simulink model "BASIC_PRACTICES"  (R2025a)
settings: Solver=FixedStepDiscrete  StartTime=0.0  StopTime=10.0  FixedStep=.5  RelTol=1e-3
libraries: simulink x15, simulink_extras x1, SignalEditorBlockLib x1
settings Model: Creator=shubh  LastModifiedBy=shubh

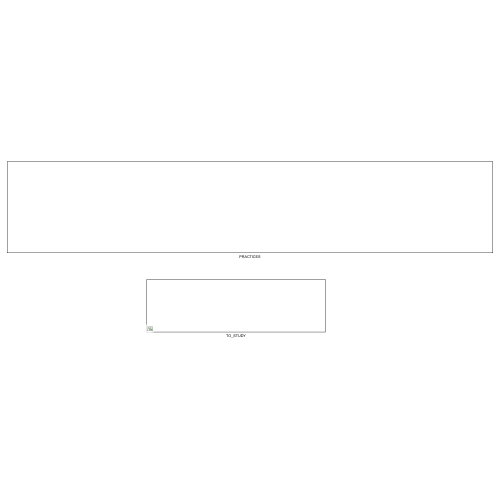
[thumbnail: Simulink's stored preview of the top-level diagram]
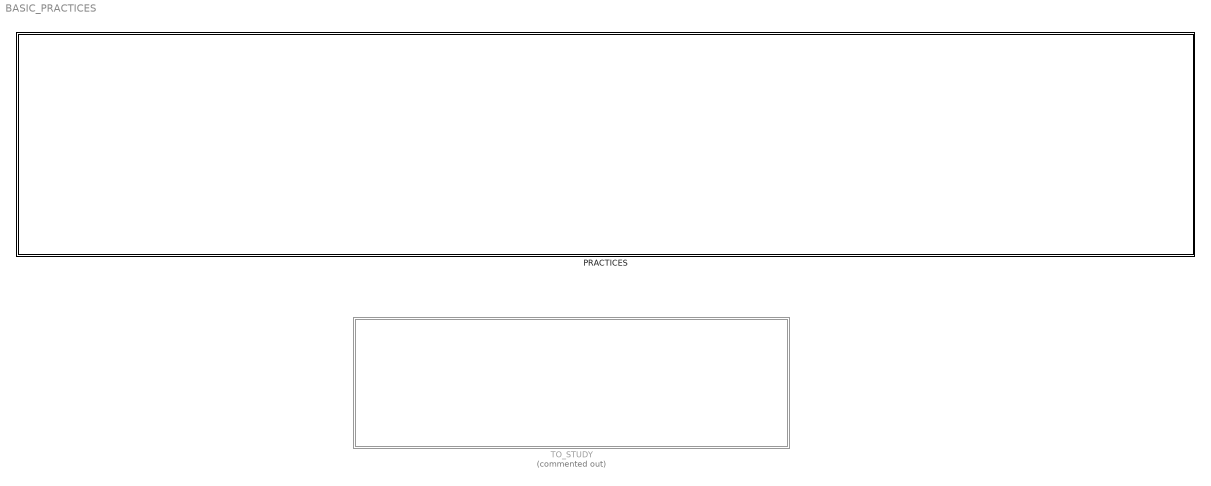
== system BASIC_PRACTICES ==
  PRACTICES : Subsystem
  TO_STUDY : Subsystem  Commented=on

== system BASIC_PRACTICES/PRACTICES ==
  Simulink : Subsystem  Commented=on
  Stateflow : Subsystem  Commented=on
  Subsystem : Subsystem  Commented=on

== system BASIC_PRACTICES/TO_STUDY ==
  Chart : Stateflow chart  TreatAsAtomicUnit=on
  Signal Editor : SignalEditorBlockLib/Signal Editor  FileName=untitled.mat  ActiveScenario=Scenario  ActiveSignal=Signal 1  IsBus=off  OutputBusObjectStr=Bus: BusObject  SampleTime=0  Interpolate=off  ZeroCross=off  OutputAfterFinalValue=Setting to zero  Unit=inherit  PreserveSignalName=on  ApplySigPropsToAllScenarios=on  ApplySigPropsToAllSignals=off  SignalPropertySource=Dialog parameters

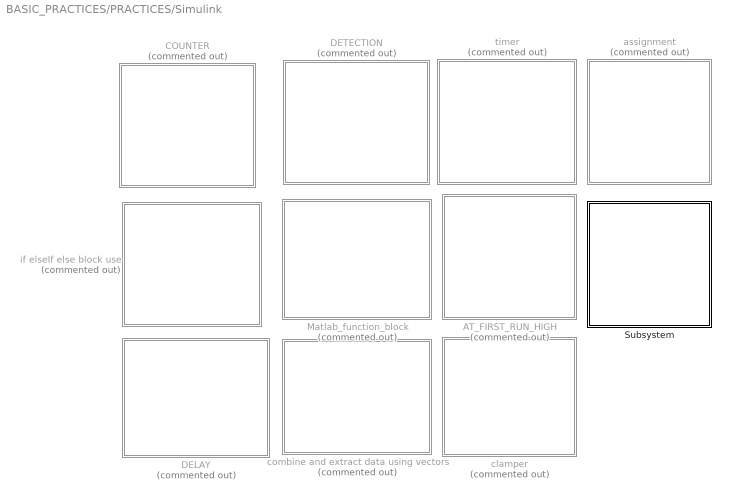
== system BASIC_PRACTICES/PRACTICES/Simulink ==
  AT_FIRST_RUN_HIGH : Subsystem  Commented=on
  COUNTER : Subsystem  Commented=on
  DELAY : Subsystem  Commented=on
  DETECTION : Subsystem  Commented=on
  Matlab_function_block : Subsystem  Commented=on
  Subsystem : Subsystem
  assignment : Subsystem  Commented=on
  clamper : Subsystem  Commented=on
  combine and extract data using vectors : Subsystem  Commented=on
  if elseIf else block use : Subsystem  Commented=on
  timer : Subsystem  Commented=on

== system BASIC_PRACTICES/PRACTICES/Stateflow ==
  For_loop : Subsystem  Commented=on
  counter : Subsystem  Commented=on
  delay_wo_delay_block : Subsystem  Commented=on
  if_else : Subsystem  Commented=on

== system BASIC_PRACTICES/PRACTICES/Subsystem ==
  BY_MATLAB_function : Subsystem  Commented=on
  Subsystem : Subsystem

== system BASIC_PRACTICES/TO_STUDY/Chart/? ==
  Action Port : ActionPort
      settings: CopyFcn=Stateflow.SLINSF.SimulinkMan.removeBlockPreDeleteFcn  PreDeleteFcn=Stateflow.SLINSF.SimulinkMan.unsafePredeleteFcn

== system BASIC_PRACTICES/TO_STUDY/Chart/?1 ==
  Action Port : ActionPort
      settings: CopyFcn=Stateflow.SLINSF.SimulinkMan.removeBlockPreDeleteFcn  PreDeleteFcn=Stateflow.SLINSF.SimulinkMan.unsafePredeleteFcn

== system BASIC_PRACTICES/TO_STUDY/Chart/?2 ==
  f : TriggerPort  TriggerType=function-call  VariantControl=(inherit)
      settings: CopyFcn=Stateflow.SLINSF.SimulinkMan.removeBlockPreDeleteFcn  PreDeleteFcn=Stateflow.SLINSF.SimulinkMan.unsafePredeleteFcn

== system BASIC_PRACTICES/PRACTICES/Simulink/AT_FIRST_RUN_HIGH ==
  AND : Logic  IconShape=distinctive  AllPortsSameDT=off  OutDataTypeStr=boolean
  Constant : Constant  OutDataTypeStr=boolean
  Pulse Generator : DiscretePulseGenerator  PulseType=Time based  Amplitude=2  PulseWidth=50  PhaseDelay=1
  Scope : Scope  NumInputPorts=2
      settings: ActiveDisplayYMinimum=-1  ActiveDisplayYMaximum=1
  Switch : Switch  Criteria=u2 > Threshold  SaturateOnIntegerOverflow=off  InputSameDT=off
  Unit Delay : UnitDelay  SampleTime=-1  HasFrameUpgradeWarning=on
  wires:
  Constant/1 -> AND/1
  Switch/1 -> Unit Delay/1, Scope/1
  Pulse Generator/1 -> Scope/2, AND/2
  AND/1 -> Switch/1, Switch/2
  Unit Delay/1 -> Switch/3

== system BASIC_PRACTICES/PRACTICES/Simulink/COUNTER ==
  DOWN : Subsystem
  UP_DOWN : Subsystem
  enabled_and_reset : Subsystem
  up : Subsystem

== system BASIC_PRACTICES/PRACTICES/Simulink/DELAY ==
  OFF_DELAY_WITH_BASIC_BLOCKS : Subsystem
  ON_DELAY_WITH_BASIC_BLOCKS : Subsystem
  ON_OFF_DELAY_ONE_STEP : Subsystem

== system BASIC_PRACTICES/PRACTICES/Simulink/DETECTION ==
  EDGE_DETECTION : Subsystem
  HYSTERESIS : Subsystem
  OUT_OF_RANGE_DETECTION : Subsystem
  max-of-three-input : Subsystem

== system BASIC_PRACTICES/PRACTICES/Simulink/Matlab_function_block ==
  MATLAB Function : MATLAB Function  TreatAsAtomicUnit=on
  Repeating Sequence Stair : simulink/Sources/Repeating Sequence Stair  OutValues=[1 -2 2 3].'  tsamp=-1  OutMin=[]  OutMax=[]  OutDataTypeStr=double  OutputDataTypeScalingMode=double  OutDataType=fixdt(0,8)  ConRadixGroup=Best Precision: Vector-wise  OutScaling=2^-12
  Scope : Scope  NumInputPorts=2
      settings: ActiveDisplayYMinimum=-2.625  ActiveDisplayYMaximum=3.625  DataLoggingVariableName=ScopeData2
  wires:
  MATLAB Function/1(y) -> Scope/2
  Repeating Sequence Stair/1 -> Scope/1, MATLAB Function/1(u)

== system BASIC_PRACTICES/PRACTICES/Simulink/Subsystem ==

== system BASIC_PRACTICES/PRACTICES/Simulink/assignment ==
  Assignment : Assignment  DiagnosticForDimensions=Warning  IndexOptions=Starting index (port)  Indices=[2 ]  OutputSizes=5
  Constant : Constant  Value=[0 0 0 0 0]
  Display : Display
  Repeating Sequence Stair : simulink/Sources/Repeating Sequence Stair  OutValues=[5 4 3 2 1].'  tsamp=-1  OutMin=[]  OutMax=[]  OutDataTypeStr=double  OutputDataTypeScalingMode=double  OutDataType=fixdt(0,8)  ConRadixGroup=Best Precision: Vector-wise  OutScaling=2^-12
  Repeating Sequence Stair1 : simulink/Sources/Repeating Sequence Stair  OutValues=[1 2 3 4 5].'  tsamp=-1  OutMin=[]  OutMax=[]  OutDataTypeStr=double  OutputDataTypeScalingMode=double  OutDataType=fixdt(0,8)  ConRadixGroup=Best Precision: Vector-wise  OutScaling=2^-12
  wires:
  Constant/1 -> Assignment/1
  Repeating Sequence Stair/1 -> Assignment/2
  Assignment/1 -> Display/1
  Repeating Sequence Stair1/1 -> Assignment/3

== system BASIC_PRACTICES/PRACTICES/Simulink/clamper ==
  Add : Sum
  Constant : Constant
  Repeating Sequence Stair : simulink/Sources/Repeating Sequence Stair  OutValues=[-5 5].'  tsamp=-1  OutMin=[]  OutMax=[]  OutDataTypeStr=double  OutputDataTypeScalingMode=double  OutDataType=fixdt(0,8)  ConRadixGroup=Best Precision: Vector-wise  OutScaling=2^-12
  Scope : Scope  NumInputPorts=2
      settings: ActiveDisplayYMinimum=-6.25  ActiveDisplayYMaximum=6.25  DataLoggingVariableName=ScopeData2
  wires:
  Add/1 -> Scope/2
  Repeating Sequence Stair/1 -> Scope/1, Add/1
  Constant/1 -> Add/2

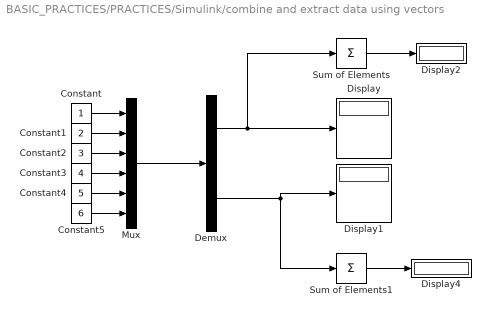
== system BASIC_PRACTICES/PRACTICES/Simulink/combine and extract data using vectors ==
  Constant : Constant
  Constant1 : Constant  Value=2
  Constant2 : Constant  Value=3
  Constant3 : Constant  Value=4
  Constant4 : Constant  Value=5
  Constant5 : Constant  Value=6
  Demux : Demux  Outputs=2
  Display{,1..2,4} (4 alike) : Display
  Mux : Mux  Inputs=6
  Sum of Elements : Sum  Inputs=+
  Sum of Elements1 : Sum  Inputs=+
  wires:
  Mux/1 -> Demux/1
  Constant5/1 -> Mux/6
  Constant4/1 -> Mux/5
  Constant3/1 -> Mux/4
  Constant2/1 -> Mux/3
  Constant1/1 -> Mux/2
  Constant/1 -> Mux/1
  Demux/1 -> Sum of Elements/1, Display/1
  Demux/2 -> Display1/1, Sum of Elements1/1
  Sum of Elements/1 -> Display2/1
  Sum of Elements1/1 -> Display4/1

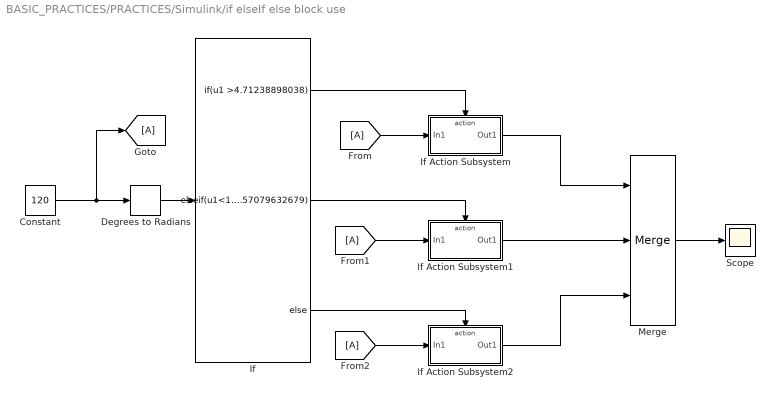
== system BASIC_PRACTICES/PRACTICES/Simulink/if elseIf else block use ==
  Constant : Constant  Value=120  OutDataTypeStr=Inherit: Inherit via back propagation
  Degrees to Radians : simulink_extras/Transformations/Degrees to Radians
  From : From
  From1 : From
  From2 : From
  Goto : Goto
  If : If  IfExpression=u1 >4.71238898038  ElseIfExpressions=u1<1.57079632679
  If Action Subsystem : Subsystem  TreatAsAtomicUnit=on
  If Action Subsystem1 : Subsystem  TreatAsAtomicUnit=on
  If Action Subsystem2 : Subsystem  TreatAsAtomicUnit=on
  Merge : Merge  Inputs=3
  Scope : Scope
      settings: ActiveDisplayYMinimum=0.48061  ActiveDisplayYMaximum=0.68061
  wires:
  Constant/1 -> Degrees to Radians/1, Goto/1
  Merge/1 -> Scope/1
  From/1 -> If Action Subsystem/1(In1)
  From1/1 -> If Action Subsystem1/1(In1)
  From2/1 -> If Action Subsystem2/1(In1)
  If/3 -> If Action Subsystem2/Action
  If/2 -> If Action Subsystem1/Action
  If/1 -> If Action Subsystem/Action
  If Action Subsystem/1(Out1) -> Merge/1
  If Action Subsystem1/1(Out1) -> Merge/2
  If Action Subsystem2/1(Out1) -> Merge/3
  Degrees to Radians/1 -> If/1

== system BASIC_PRACTICES/PRACTICES/Simulink/timer ==
  Counting_1_MINUTE : Subsystem  Commented=on
  OFF_DELAY_WITH_BASIC_BLOCKS : Subsystem  Commented=on
  ON_DELAY_WITH_BASIC_BLOCKS : Subsystem  Commented=on
  ON_OFF_DELAY_ONE_STEP : Subsystem  Commented=on

== system BASIC_PRACTICES/PRACTICES/Stateflow/For_loop ==
  Chart : Stateflow chart  TreatAsAtomicUnit=on
  Chart1 : Stateflow chart  TreatAsAtomicUnit=on
  Repeating Sequence Stair : simulink/Sources/Repeating Sequence Stair  OutValues=[0 1].'  tsamp=-1  OutMin=[]  OutMax=[]  OutDataTypeStr=double  OutputDataTypeScalingMode=double  OutDataType=fixdt(0,8)  ConRadixGroup=Best Precision: Vector-wise  OutScaling=2^-12
  Scope : Scope  NumInputPorts=2
      settings: ActiveDisplayYMinimum=45  ActiveDisplayYMaximum=65  DataLoggingVariableName=ScopeData2
  wires:
  Chart1/1(out) -> Scope/1
  Chart/1(out) -> Scope/2
  Repeating Sequence Stair/1 -> Chart/1(en)

== system BASIC_PRACTICES/PRACTICES/Stateflow/counter ==
  Chart : Stateflow chart  TreatAsAtomicUnit=on
  Scope : Scope
      settings: ActiveDisplayYMinimum=-0.625  ActiveDisplayYMaximum=5.625  DataLoggingVariableName=ScopeData4
  wires:
  Chart/1(z) -> Scope/1

== system BASIC_PRACTICES/PRACTICES/Stateflow/delay_wo_delay_block ==
  Chart : Stateflow chart  TreatAsAtomicUnit=on
      settings: PortSchema="{\"entries\":[{\"content\":{\"sides\":[{\"content\":{\"connectorIds\":[\"In4\",\"In1\",\"In2\",\"In3\"]},\"type\":\"ConnectorPlacement.EquallySpacedRectSide\",\"uuid\":\"e0e5e045-d7b2-46b3-b410-3be38740735a\"},{\"content\":{\"connectorIds\":[\"Out1\",\"Out2\"],\"side\":\"RIGHT\"},\"type\":\"ConnectorPlacement.EquallySpacedRectSide\",\"uuid\":\"4f12564d-9a97-4df6-80a9-b07c0bfc5d80\"},{\"content\":{\"side\":\"TOP\"},\"type\":\"ConnectorPlacement.EquallySpacedRectSide\",\"uuid\":\"29280d5c-fd79-4991-91bd-bd3cbc2b5a83\"}]},\"type\":\"ConnectorPlacement.EquallySpacedConnector\",\"uuid\":\"51515ad8-eb0a-4d19-8f24-8c6bcb3a19d7\"}],\"packageUris\":[\"http://schema.mathworks.com/mf0/Connector/R2020b\"],\"version\":\"1.0\"}"
  Constant : Constant  OutDataTypeStr=uint16
  Counter Free-Running : simulink/Sources/Counter Free-Running  NumBits=16  tsamp=-1
  Data Store Memory : DataStoreMemory  WriteAfterWriteMsg=warning  ShowAdditionalParam=off
  Data Store Read : DataStoreRead  IndexOptions=Index vector (dialog)  Indices=1  OutputSizes=1
  Data Store Write1 : DataStoreWrite  IndexOptions=Index vector (dialog)  Indices=1  OutputSizes=1
  Repeating Sequence Stair : simulink/Sources/Repeating Sequence Stair  OutValues=[3 1 2].'  tsamp=-1  OutMin=[]  OutMax=[]  OutDataTypeStr=uint16  OutputDataTypeScalingMode=uint16  OutDataType=fixdt(0,8)  ConRadixGroup=Best Precision: Vector-wise  OutScaling=2^-12
  Scope : Scope  NumInputPorts=3
      settings: ActiveDisplayYMinimum=0.75  ActiveDisplayYMaximum=3.25
  wires:
  Counter Free-Running/1 -> Chart/3(t)
  Repeating Sequence Stair/1 -> Chart/4(in), Scope/1
  Constant/1 -> Chart/1(inVal)
  Data Store Read/1 -> Chart/2(oldIn)
  Chart/2(oldValue) -> Scope/3, Data Store Write1/1
  Chart/1(out) -> Scope/2

== system BASIC_PRACTICES/PRACTICES/Stateflow/if_else ==
  Chart : Stateflow chart  TreatAsAtomicUnit=on
  Constant : Constant
  Scope : Scope
      settings: DataLoggingVariableName=ScopeData3
  wires:
  Chart/1(y) -> Scope/1
  Constant/1 -> Chart/1(h)

== system BASIC_PRACTICES/PRACTICES/Subsystem/BY_MATLAB_function ==
  Constant : Constant  Value=5
  Display : Display
  MATLAB Function : MATLAB Function  TreatAsAtomicUnit=on
  wires:
  Constant/1 -> MATLAB Function/1(n)
  MATLAB Function/1(y) -> Display/1

== system BASIC_PRACTICES/PRACTICES/Subsystem/Subsystem ==
  note: run 1 step for correct
      | output
  Constant : Constant  Value=5
  Display : Display
  For Iterator Subsystem : Subsystem  TreatAsAtomicUnit=on
  wires:
  Constant/1 -> For Iterator Subsystem/1(In2)
  For Iterator Subsystem/1(Out1) -> Display/1

== system BASIC_PRACTICES/PRACTICES/Simulink/COUNTER/DOWN ==
  Add : Sum  Inputs=-+
  Compare To Constant : simulink/Logic and Bit Operations/Compare To Constant  relop=<=  const=0  OutDataTypeStr=boolean
  Constant : Constant
  Constant2 : Constant  Value=5
  Scope : Scope
      settings: ActiveDisplayYMinimum=-24.56203  ActiveDisplayYMaximum=9.14991
  Switch : Switch  Criteria=u2 > Threshold  SaturateOnIntegerOverflow=off  InputSameDT=off
  Unit Delay : UnitDelay  InitialCondition=6  SampleTime=-1  HasFrameUpgradeWarning=on
  wires:
  Constant/1 -> Add/1
  Add/1 -> Switch/3, Compare To Constant/1
  Unit Delay/1 -> Add/2
  Switch/1 -> Unit Delay/1, Scope/1
  Compare To Constant/1 -> Switch/2
  Constant2/1 -> Switch/1

== system BASIC_PRACTICES/PRACTICES/Simulink/COUNTER/UP_DOWN ==

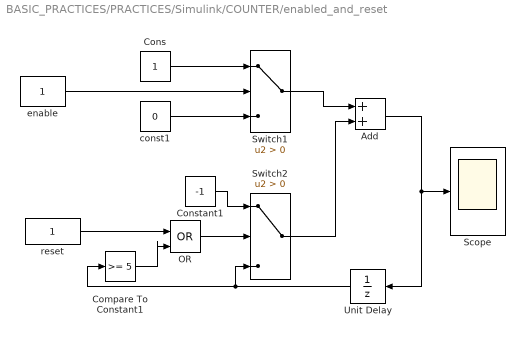
== system BASIC_PRACTICES/PRACTICES/Simulink/COUNTER/enabled_and_reset ==
  Add : Sum
  Compare To Constant1 : simulink/Logic and Bit Operations/Compare To Constant  relop=>=  const=5  OutDataTypeStr=boolean
  Cons : Constant
  Constant1 : Constant  Value=-1
  OR : Logic  Operator=OR  IconShape=distinctive  AllPortsSameDT=off  OutDataTypeStr=boolean
  Scope : Scope
      settings: ActiveDisplayYMinimum=-0.625  ActiveDisplayYMaximum=5.625
  Switch1 : Switch  Criteria=u2 > Threshold  SaturateOnIntegerOverflow=off  InputSameDT=off
  Switch2 : Switch  Criteria=u2 > Threshold  SaturateOnIntegerOverflow=off  InputSameDT=off
  Unit Delay : UnitDelay  InitialCondition=-1  SampleTime=-1  HasFrameUpgradeWarning=on
  const1 : Constant  Value=0
  enable : Constant
  reset : Constant
  wires:
  Add/1 -> Unit Delay/1, Scope/1
  Unit Delay/1 -> Compare To Constant1/1, Switch2/3
  Switch1/1 -> Add/1
  const1/1 -> Switch1/3
  Cons/1 -> Switch1/1
  enable/1 -> Switch1/2
  Switch2/1 -> Add/2
  reset/1 -> OR/1
  Constant1/1 -> Switch2/1
  Compare To Constant1/1 -> OR/2
  OR/1 -> Switch2/2

== system BASIC_PRACTICES/PRACTICES/Simulink/COUNTER/up ==
  Add : Sum
  Compare To Constant : simulink/Logic and Bit Operations/Compare To Constant  relop=<=  const=5  OutDataTypeStr=boolean
  Constant : Constant
  Constant1 : Constant  Value=0
  Scope1 : Scope
      settings: ActiveDisplayYMinimum=-0.625  ActiveDisplayYMaximum=5.625  DataLoggingVariableName=ScopeData2
  Switch : Switch  Criteria=u2 > Threshold  SaturateOnIntegerOverflow=off  InputSameDT=off
  Unit Delay : UnitDelay  InitialCondition=-1  SampleTime=-1  HasFrameUpgradeWarning=on
  wires:
  Switch/1 -> Scope1/1, Unit Delay/1
  Add/1 -> Switch/1, Compare To Constant/1
  Compare To Constant/1 -> Switch/2
  Constant/1 -> Add/1
  Constant1/1 -> Switch/3
  Unit Delay/1 -> Add/2

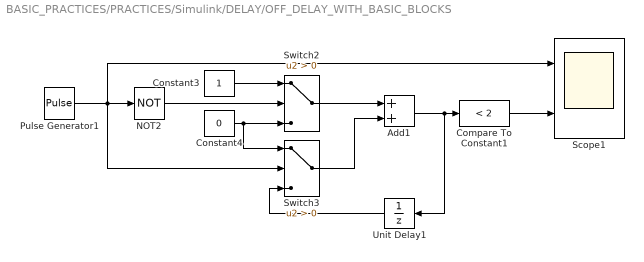
== system BASIC_PRACTICES/PRACTICES/Simulink/DELAY/OFF_DELAY_WITH_BASIC_BLOCKS ==
  Add1 : Sum
  Compare To Constant1 : simulink/Logic and Bit Operations/Compare To Constant  relop=<  const=2  OutDataTypeStr=boolean
  Constant3 : Constant
  Constant4 : Constant  Value=0
  NOT2 : Logic  Operator=NOT  IconShape=distinctive  AllPortsSameDT=off  OutDataTypeStr=boolean
  Pulse Generator1 : DiscretePulseGenerator  PulseType=Time based  PulseWidth=50  PhaseDelay=.5
  Scope1 : Scope  NumInputPorts=2
      settings: ActiveDisplayYMinimum=-0.125  ActiveDisplayYMaximum=1.125  DataLoggingVariableName=ScopeData3
  Switch2 : Switch  Criteria=u2 > Threshold  SaturateOnIntegerOverflow=off  InputSameDT=off
  Switch3 : Switch  Criteria=u2 > Threshold  SaturateOnIntegerOverflow=off  InputSameDT=off
  Unit Delay1 : UnitDelay  SampleTime=-1  HasFrameUpgradeWarning=on
  wires:
  Switch3/1 -> Add1/2
  NOT2/1 -> Switch2/2
  Unit Delay1/1 -> Switch3/3
  Add1/1 -> Unit Delay1/1, Compare To Constant1/1
  Compare To Constant1/1 -> Scope1/2
  Constant4/1 -> Switch3/1, Switch2/3
  Pulse Generator1/1 -> Switch3/2, NOT2/1, Scope1/1
  Constant3/1 -> Switch2/1
  Switch2/1 -> Add1/1

== system BASIC_PRACTICES/PRACTICES/Simulink/DELAY/ON_DELAY_WITH_BASIC_BLOCKS ==
  note: RISING_DELAY_0.5sec_SOLVER=.25
  Add1 : Sum
  Compare To Constant1 : simulink/Logic and Bit Operations/Compare To Constant  relop=>=  const=.75  OutDataTypeStr=boolean
  Constant3 : Constant  Value=.25
  Constant4 : Constant  Value=0
  NOT1 : Logic  Operator=NOT  IconShape=distinctive  AllPortsSameDT=off  OutDataTypeStr=boolean
  Pulse Generator1 : DiscretePulseGenerator  PulseType=Time based  PulseWidth=50  PhaseDelay=.5
  Scope1 : Scope  NumInputPorts=2
      settings: ActiveDisplayYMinimum=-0.125  ActiveDisplayYMaximum=1.125  DataLoggingVariableName=ScopeData6
  Switch2 : Switch  Criteria=u2 > Threshold  SaturateOnIntegerOverflow=off  InputSameDT=off
  Switch3 : Switch  Criteria=u2 > Threshold  SaturateOnIntegerOverflow=off  InputSameDT=off
  Unit Delay1 : UnitDelay  SampleTime=-1  HasFrameUpgradeWarning=on
  wires:
  NOT1/1 -> Switch3/2
  Switch3/1 -> Add1/2
  Constant3/1 -> Switch2/1
  Switch2/1 -> Add1/1
  Add1/1 -> Unit Delay1/1, Compare To Constant1/1
  Compare To Constant1/1 -> Scope1/2
  Unit Delay1/1 -> Switch3/3
  Pulse Generator1/1 -> NOT1/1, Switch2/2, Scope1/1
  Constant4/1 -> Switch3/1, Switch2/3

== system BASIC_PRACTICES/PRACTICES/Simulink/DELAY/ON_OFF_DELAY_ONE_STEP ==
  OFF_DELAY : Subsystem  Commented=on
  ON_DELAY : Subsystem  Commented=on

== system BASIC_PRACTICES/PRACTICES/Simulink/DETECTION/EDGE_DETECTION ==
  FALLING : Subsystem  Commented=on
  FALLING_EDGE_COUNT : Subsystem  Commented=on
  Rising : Subsystem  Commented=on
  Rising_EDGE_COUNT : Subsystem  Commented=on
  rising_falling_edge_detection_and_counting : Subsystem  Commented=on

== system BASIC_PRACTICES/PRACTICES/Simulink/DETECTION/HYSTERESIS ==
  BLOCK : Subsystem  Commented=on
  HYSTERESIS : Subsystem  Commented=on
  REVERSE_HYSTERESIS : Subsystem  Commented=on

== system BASIC_PRACTICES/PRACTICES/Simulink/DETECTION/OUT_OF_RANGE_DETECTION ==
  AND1 : Logic  Operator=OR  IconShape=distinctive  AllPortsSameDT=off  OutDataTypeStr=boolean
  Constant : Constant  Value=2
  Constant1 : Constant  Value=-2
  Constant2 : Constant  OutDataTypeStr=boolean
  Constant3 : Constant  Value=0  OutDataTypeStr=boolean
  GreaterThan : RelationalOperator  Operator=>  OutDataTypeStr=boolean  RndMeth=Simplest  InputSameDT=off
  GreaterThan1 : RelationalOperator  Operator=<  OutDataTypeStr=boolean  RndMeth=Simplest  InputSameDT=off
  Scope1 : Scope  NumInputPorts=2
      settings: ActiveDisplayYMinimum=-3.73705  ActiveDisplayYMaximum=3.74854
  Sine Wave1 : Sin  Amplitude=3  Frequency=3  SampleTime=0
  Switch : Switch  Criteria=u2 > Threshold  SaturateOnIntegerOverflow=off  InputSameDT=off
  wires:
  GreaterThan1/1 -> AND1/2
  Sine Wave1/1 -> GreaterThan1/1, GreaterThan/1, Scope1/1
  Constant/1 -> GreaterThan/2
  Constant3/1 -> Switch/3
  Constant1/1 -> GreaterThan1/2
  GreaterThan/1 -> AND1/1
  AND1/1 -> Switch/2
  Constant2/1 -> Switch/1
  Switch/1 -> Scope1/2

== system BASIC_PRACTICES/PRACTICES/Simulink/DETECTION/max-of-three-input ==
  A : Constant  Value=56
  B : Constant  Value=45
  C : Constant  Value=46
  Display1 : Display
  GreaterThan : RelationalOperator  Operator=>  OutDataTypeStr=boolean  RndMeth=Simplest  InputSameDT=off
  GreaterThanC : RelationalOperator  Operator=>  OutDataTypeStr=boolean  RndMeth=Simplest  InputSameDT=off
  Switch : Switch  Criteria=u2 > Threshold  SaturateOnIntegerOverflow=off  InputSameDT=off
  Switch1 : Switch  Criteria=u2 > Threshold  SaturateOnIntegerOverflow=off  InputSameDT=off
  wires:
  B/1 -> GreaterThan/2, Switch/3
  A/1 -> GreaterThan/1, Switch/1
  GreaterThan/1 -> Switch/2
  Switch/1 -> GreaterThanC/1, Switch1/1
  C/1 -> GreaterThanC/2, Switch1/3
  GreaterThanC/1 -> Switch1/2
  Switch1/1 -> Display1/1

== system BASIC_PRACTICES/PRACTICES/Simulink/if elseIf else block use/If Action Subsystem ==
  In1 : Inport
  Action Port : ActionPort  ActionPortLabel=if(u1 >4.71238898038)
  Multiply : Gain  Gain=0
  Out1 : Outport
  wires:
  In1/1 -> Multiply/1
  Multiply/1 -> Out1/1

== system BASIC_PRACTICES/PRACTICES/Simulink/if elseIf else block use/If Action Subsystem1 ==
  In1 : Inport
  Action Port : ActionPort  ActionPortLabel=elseif(u1<1.57079632679)
  Multiply : Gain  Gain=0
  Out1 : Outport
  wires:
  In1/1 -> Multiply/1
  Multiply/1 -> Out1/1

== system BASIC_PRACTICES/PRACTICES/Simulink/if elseIf else block use/If Action Subsystem2 ==
  In1 : Inport
  Action Port : ActionPort  ActionPortLabel=else
  Sinh1 : Trigonometry
  Out1 : Outport
  wires:
  Sinh1/1 -> Out1/1
  In1/1 -> Sinh1/1

== system BASIC_PRACTICES/PRACTICES/Simulink/timer/Counting_1_MINUTE ==
  Add1 : Sum
  Constant2 : Constant
  Constant3 : Constant  Value=61
  GreaterThan1 : RelationalOperator  Operator===  OutDataTypeStr=boolean  RndMeth=Simplest  InputSameDT=off
  Scope1 : Scope
      settings: ActiveDisplayYMinimum=-0.125  ActiveDisplayYMaximum=1.125  DataLoggingVariableName=ScopeData6
  Unit Delay1 : UnitDelay  SampleTime=-1  HasFrameUpgradeWarning=on
  wires:
  Add1/1 -> Unit Delay1/1, GreaterThan1/1
  GreaterThan1/1 -> Scope1/1
  Constant2/1 -> Add1/1
  Unit Delay1/1 -> Add1/2
  Constant3/1 -> GreaterThan1/2

== system BASIC_PRACTICES/PRACTICES/Simulink/timer/OFF_DELAY_WITH_BASIC_BLOCKS ==
  Add1 : Sum
  Compare To Constant1 : simulink/Logic and Bit Operations/Compare To Constant  relop=<  const=2  OutDataTypeStr=boolean
  Constant3 : Constant
  Constant4 : Constant  Value=0
  NOT2 : Logic  Operator=NOT  IconShape=distinctive  AllPortsSameDT=off  OutDataTypeStr=boolean
  Pulse Generator1 : DiscretePulseGenerator  PulseType=Time based  PulseWidth=50  PhaseDelay=.5
  Scope1 : Scope  NumInputPorts=2
      settings: ActiveDisplayYMinimum=-0.125  ActiveDisplayYMaximum=1.125  DataLoggingVariableName=ScopeData3
  Switch2 : Switch  Criteria=u2 > Threshold  SaturateOnIntegerOverflow=off  InputSameDT=off
  Switch3 : Switch  Criteria=u2 > Threshold  SaturateOnIntegerOverflow=off  InputSameDT=off
  Unit Delay1 : UnitDelay  SampleTime=-1  HasFrameUpgradeWarning=on
  wires:
  Switch3/1 -> Add1/2
  NOT2/1 -> Switch2/2
  Unit Delay1/1 -> Switch3/3
  Add1/1 -> Unit Delay1/1, Compare To Constant1/1
  Compare To Constant1/1 -> Scope1/2
  Constant4/1 -> Switch3/1, Switch2/3
  Pulse Generator1/1 -> Switch3/2, NOT2/1, Scope1/1
  Constant3/1 -> Switch2/1
  Switch2/1 -> Add1/1

== system BASIC_PRACTICES/PRACTICES/Simulink/timer/ON_DELAY_WITH_BASIC_BLOCKS ==
  note: RISING_DELAY_0.5sec_SOLVER=.25
  Add1 : Sum
  Compare To Constant1 : simulink/Logic and Bit Operations/Compare To Constant  relop=>=  const=.75  OutDataTypeStr=boolean
  Constant3 : Constant  Value=.25
  Constant4 : Constant  Value=0
  NOT1 : Logic  Operator=NOT  IconShape=distinctive  AllPortsSameDT=off  OutDataTypeStr=boolean
  Pulse Generator1 : DiscretePulseGenerator  PulseType=Time based  PulseWidth=50  PhaseDelay=.5
  Scope1 : Scope  NumInputPorts=2
      settings: ActiveDisplayYMinimum=-0.125  ActiveDisplayYMaximum=1.125  DataLoggingVariableName=ScopeData6
  Switch2 : Switch  Criteria=u2 > Threshold  SaturateOnIntegerOverflow=off  InputSameDT=off
  Switch3 : Switch  Criteria=u2 > Threshold  SaturateOnIntegerOverflow=off  InputSameDT=off
  Unit Delay1 : UnitDelay  SampleTime=-1  HasFrameUpgradeWarning=on
  wires:
  NOT1/1 -> Switch3/2
  Switch3/1 -> Add1/2
  Constant3/1 -> Switch2/1
  Switch2/1 -> Add1/1
  Add1/1 -> Unit Delay1/1, Compare To Constant1/1
  Compare To Constant1/1 -> Scope1/2
  Unit Delay1/1 -> Switch3/3
  Pulse Generator1/1 -> NOT1/1, Switch2/2, Scope1/1
  Constant4/1 -> Switch3/1, Switch2/3

== system BASIC_PRACTICES/PRACTICES/Simulink/timer/ON_OFF_DELAY_ONE_STEP ==
  OFF_DELAY : Subsystem  Commented=on
  ON_DELAY : Subsystem  Commented=on

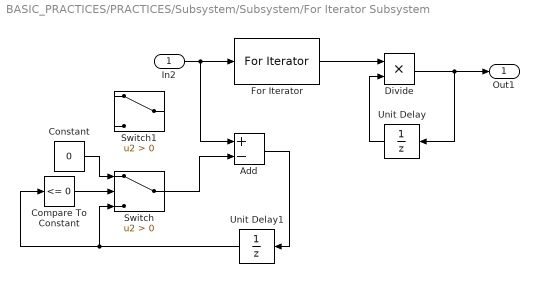
== system BASIC_PRACTICES/PRACTICES/Subsystem/Subsystem/For Iterator Subsystem ==
  In2 : Inport
  Add : Sum  Inputs=+-
  Compare To Constant : simulink/Logic and Bit Operations/Compare To Constant  relop=<=  const=0  OutDataTypeStr=boolean
  Constant : Constant  Value=0
  Divide : Product  Inputs=**
  For Iterator : ForIterator  IterationSource=external  IterationVariableDataType=double
  Switch : Switch  Criteria=u2 > Threshold  SaturateOnIntegerOverflow=off  InputSameDT=off
  Switch1 : Switch  Criteria=u2 > Threshold  SaturateOnIntegerOverflow=off  InputSameDT=off
  Unit Delay : UnitDelay  InitialCondition=1  SampleTime=-1  HasFrameUpgradeWarning=on
  Unit Delay1 : UnitDelay  InitialCondition=1  SampleTime=-1  HasFrameUpgradeWarning=on
  Out1 : Outport
  wires:
  In2/1 -> Add/1, For Iterator/1
  For Iterator/1 -> Divide/1
  Divide/1 -> Unit Delay/1, Out1/1
  Unit Delay/1 -> Divide/2
  Add/1 -> Unit Delay1/1
  Unit Delay1/1 -> Switch/3, Compare To Constant/1
  Switch/1 -> Add/2
  Compare To Constant/1 -> Switch/2
  Constant/1 -> Switch/1

== system BASIC_PRACTICES/PRACTICES/Simulink/DELAY/ON_OFF_DELAY_ONE_STEP/OFF_DELAY ==
  Constant1 : Constant
  GreaterThan : RelationalOperator  Operator=<  OutDataTypeStr=boolean  RndMeth=Simplest  InputSameDT=off
  Pulse Generator : DiscretePulseGenerator  PulseType=Time based  PulseWidth=50  PhaseDelay=1
  Scope : Scope  NumInputPorts=2
      settings: ActiveDisplayYMinimum=-0.125  ActiveDisplayYMaximum=1.125
  Switch : Switch  Criteria=u2 > Threshold  SaturateOnIntegerOverflow=off  InputSameDT=off
  Unit Delay1 : UnitDelay  SampleTime=-1  HasFrameUpgradeWarning=on
  wires:
  Constant1/1 -> GreaterThan/2
  Switch/1 -> Scope/2
  GreaterThan/1 -> Switch/2
  Pulse Generator/1 -> Scope/1, Unit Delay1/1, Switch/3, GreaterThan/1
  Unit Delay1/1 -> Switch/1

== system BASIC_PRACTICES/PRACTICES/Simulink/DELAY/ON_OFF_DELAY_ONE_STEP/ON_DELAY ==
  Constant1 : Constant
  GreaterThan : RelationalOperator  Operator=<  OutDataTypeStr=boolean  RndMeth=Simplest  InputSameDT=off
  Pulse Generator : DiscretePulseGenerator  PulseType=Time based  PulseWidth=50  PhaseDelay=1
  Scope : Scope  NumInputPorts=2
      settings: ActiveDisplayYMinimum=-0.125  ActiveDisplayYMaximum=1.125  DataLoggingVariableName=ScopeData5
  Switch : Switch  Criteria=u2 > Threshold  SaturateOnIntegerOverflow=off  InputSameDT=off
  Unit Delay : UnitDelay  SampleTime=-1  HasFrameUpgradeWarning=on
  wires:
  Pulse Generator/1 -> Scope/1, Switch/1, Unit Delay/1, GreaterThan/1
  Constant1/1 -> GreaterThan/2
  Unit Delay/1 -> Switch/3
  GreaterThan/1 -> Switch/2
  Switch/1 -> Scope/2

== system BASIC_PRACTICES/PRACTICES/Simulink/DETECTION/EDGE_DETECTION/FALLING ==
  AND : Logic  IconShape=distinctive  AllPortsSameDT=off  OutDataTypeStr=boolean
  NOT1 : Logic  Operator=NOT  IconShape=distinctive  AllPortsSameDT=off  OutDataTypeStr=boolean
  Pulse Generator : DiscretePulseGenerator  PulseType=Time based  PulseWidth=50  PhaseDelay=1
  Scope : Scope  NumInputPorts=2
      settings: ActiveDisplayYMinimum=-0.125  ActiveDisplayYMaximum=1.125  DataLoggingVariableName=ScopeData2
  Unit Delay2 : UnitDelay  SampleTime=-1  HasFrameUpgradeWarning=on
  wires:
  Pulse Generator/1 -> Scope/1, NOT1/1, Unit Delay2/1
  AND/1 -> Scope/2
  Unit Delay2/1 -> AND/2
  NOT1/1 -> AND/1

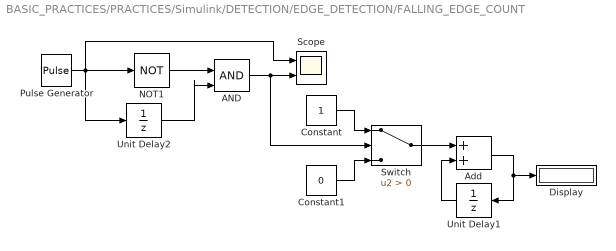
== system BASIC_PRACTICES/PRACTICES/Simulink/DETECTION/EDGE_DETECTION/FALLING_EDGE_COUNT ==
  AND : Logic  IconShape=distinctive  AllPortsSameDT=off  OutDataTypeStr=boolean
  Add : Sum
  Constant : Constant
  Constant1 : Constant  Value=0
  Display : Display
  NOT1 : Logic  Operator=NOT  IconShape=distinctive  AllPortsSameDT=off  OutDataTypeStr=boolean
  Pulse Generator : DiscretePulseGenerator  PulseType=Time based  PulseWidth=50  PhaseDelay=1
  Scope : Scope  NumInputPorts=2
      settings: ActiveDisplayYMinimum=-0.125  ActiveDisplayYMaximum=1.125  DataLoggingVariableName=ScopeData2
  Switch : Switch  Criteria=u2 > Threshold  SaturateOnIntegerOverflow=off  InputSameDT=off
  Unit Delay1 : UnitDelay  SampleTime=-1  HasFrameUpgradeWarning=on
  Unit Delay2 : UnitDelay  SampleTime=-1  HasFrameUpgradeWarning=on
  wires:
  NOT1/1 -> AND/1
  Unit Delay2/1 -> AND/2
  AND/1 -> Switch/2, Scope/2
  Pulse Generator/1 -> NOT1/1, Scope/1, Unit Delay2/1
  Constant/1 -> Switch/1
  Constant1/1 -> Switch/3
  Switch/1 -> Add/1
  Add/1 -> Display/1, Unit Delay1/1
  Unit Delay1/1 -> Add/2

== system BASIC_PRACTICES/PRACTICES/Simulink/DETECTION/EDGE_DETECTION/Rising ==
  AND : Logic  IconShape=distinctive  AllPortsSameDT=off  OutDataTypeStr=boolean
  NOT2 : Logic  Operator=NOT  IconShape=distinctive  AllPortsSameDT=off  OutDataTypeStr=boolean
  Pulse Generator : DiscretePulseGenerator  PulseType=Time based  PulseWidth=50  PhaseDelay=1
  Scope : Scope  NumInputPorts=2
      settings: ActiveDisplayYMinimum=-0.125  ActiveDisplayYMaximum=1.125
  Unit Delay2 : UnitDelay  SampleTime=-1  HasFrameUpgradeWarning=on
  wires:
  Pulse Generator/1 -> Scope/1, AND/1, Unit Delay2/1
  Unit Delay2/1 -> NOT2/1
  NOT2/1 -> AND/2
  AND/1 -> Scope/2

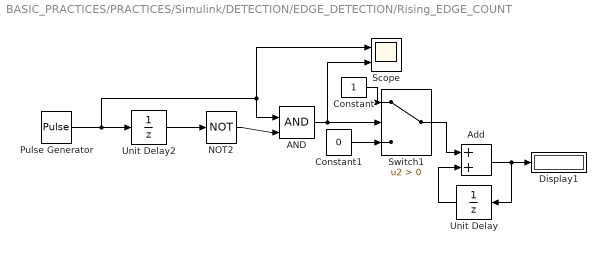
== system BASIC_PRACTICES/PRACTICES/Simulink/DETECTION/EDGE_DETECTION/Rising_EDGE_COUNT ==
  AND : Logic  IconShape=distinctive  AllPortsSameDT=off  OutDataTypeStr=boolean
  Add : Sum
  Constant : Constant
  Constant1 : Constant  Value=0
  Display1 : Display
  NOT2 : Logic  Operator=NOT  IconShape=distinctive  AllPortsSameDT=off  OutDataTypeStr=boolean
  Pulse Generator : DiscretePulseGenerator  PulseType=Time based  PulseWidth=50  PhaseDelay=1
  Scope : Scope  NumInputPorts=2
      settings: ActiveDisplayYMinimum=-0.125  ActiveDisplayYMaximum=1.125
  Switch1 : Switch  Criteria=u2 > Threshold  SaturateOnIntegerOverflow=off  InputSameDT=off
  Unit Delay : UnitDelay  SampleTime=-1  HasFrameUpgradeWarning=on
  Unit Delay2 : UnitDelay  SampleTime=-1  HasFrameUpgradeWarning=on
  wires:
  Constant1/1 -> Switch1/3
  Constant/1 -> Switch1/1
  Unit Delay2/1 -> NOT2/1
  Pulse Generator/1 -> AND/1, Scope/1, Unit Delay2/1
  AND/1 -> Scope/2, Switch1/2
  NOT2/1 -> AND/2
  Unit Delay/1 -> Add/2
  Switch1/1 -> Add/1
  Add/1 -> Unit Delay/1, Display1/1

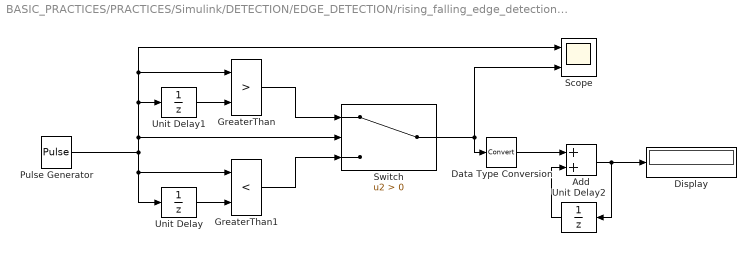
== system BASIC_PRACTICES/PRACTICES/Simulink/DETECTION/EDGE_DETECTION/rising_falling_edge_detection_and_counting ==
  Add : Sum
  Data Type Conversion : DataTypeConversion  SaturateOnIntegerOverflow=off  RndMeth=Floor
  Display : Display
  GreaterThan : RelationalOperator  Operator=>  OutDataTypeStr=boolean  RndMeth=Simplest  InputSameDT=off
  GreaterThan1 : RelationalOperator  Operator=<  OutDataTypeStr=boolean  RndMeth=Simplest  InputSameDT=off
  Pulse Generator : DiscretePulseGenerator  PulseType=Time based  Period=1  PulseWidth=50
  Scope : Scope  NumInputPorts=2
      settings: ActiveDisplayYMinimum=-0.125  ActiveDisplayYMaximum=1.125
  Switch : Switch  Criteria=u2 > Threshold  SaturateOnIntegerOverflow=off  InputSameDT=off
  Unit Delay : UnitDelay  SampleTime=-1  HasFrameUpgradeWarning=on
  Unit Delay1 : UnitDelay  SampleTime=-1  HasFrameUpgradeWarning=on
  Unit Delay2 : UnitDelay  SampleTime=-1  HasFrameUpgradeWarning=on
  wires:
  Switch/1 -> Data Type Conversion/1, Scope/2
  Pulse Generator/1 -> Unit Delay/1, GreaterThan1/1, Unit Delay1/1, GreaterThan/1, Scope/1, Switch/2
  GreaterThan/1 -> Switch/1
  Unit Delay/1 -> GreaterThan1/2
  GreaterThan1/1 -> Switch/3
  Unit Delay1/1 -> GreaterThan/2
  Add/1 -> Display/1, Unit Delay2/1
  Unit Delay2/1 -> Add/2
  Data Type Conversion/1 -> Add/1

== system BASIC_PRACTICES/PRACTICES/Simulink/DETECTION/HYSTERESIS/BLOCK ==
  Relay : Relay  OnSwitchValue=2  OffSwitchValue=-2
  Scope1 : Scope  NumInputPorts=2
      settings: ActiveDisplayYMinimum=-3.73705  ActiveDisplayYMaximum=3.74854  DataLoggingVariableName=ScopeData2
  Sine Wave : Sin  Amplitude=3  Frequency=3  SampleTime=0
  wires:
  Relay/1 -> Scope1/2
  Sine Wave/1 -> Scope1/1, Relay/1

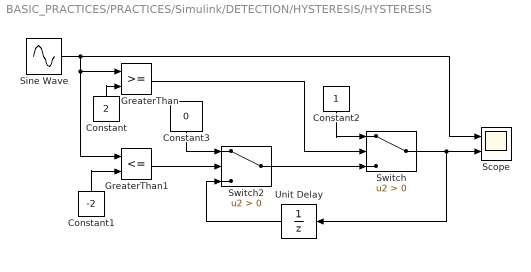
== system BASIC_PRACTICES/PRACTICES/Simulink/DETECTION/HYSTERESIS/HYSTERESIS ==
  Constant : Constant  Value=2
  Constant1 : Constant  Value=-2
  Constant2 : Constant
  Constant3 : Constant  Value=0
  GreaterThan : RelationalOperator  OutDataTypeStr=boolean  RndMeth=Simplest  InputSameDT=off
  GreaterThan1 : RelationalOperator  Operator=<=  OutDataTypeStr=boolean  RndMeth=Simplest  InputSameDT=off
  Scope : Scope  NumInputPorts=2
      settings: ActiveDisplayYMinimum=-3.73705  ActiveDisplayYMaximum=3.74854
  Sine Wave : Sin  Amplitude=3  Frequency=3  SampleTime=0
  Switch : Switch  Criteria=u2 > Threshold  SaturateOnIntegerOverflow=off  InputSameDT=off
  Switch2 : Switch  Criteria=u2 > Threshold  SaturateOnIntegerOverflow=off  InputSameDT=off
  Unit Delay : UnitDelay  SampleTime=-1  HasFrameUpgradeWarning=on
  wires:
  Sine Wave/1 -> Scope/1, GreaterThan/1, GreaterThan1/1
  GreaterThan1/1 -> Switch2/2
  GreaterThan/1 -> Switch/2
  Constant1/1 -> GreaterThan1/2
  Constant/1 -> GreaterThan/2
  Constant2/1 -> Switch/1
  Switch2/1 -> Switch/3
  Constant3/1 -> Switch2/1
  Unit Delay/1 -> Switch2/3
  Switch/1 -> Unit Delay/1, Scope/2

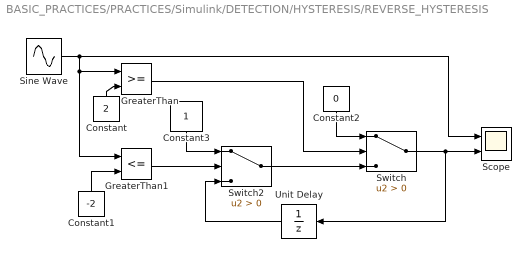
== system BASIC_PRACTICES/PRACTICES/Simulink/DETECTION/HYSTERESIS/REVERSE_HYSTERESIS ==
  Constant : Constant  Value=2
  Constant1 : Constant  Value=-2
  Constant2 : Constant  Value=0
  Constant3 : Constant
  GreaterThan : RelationalOperator  OutDataTypeStr=boolean  RndMeth=Simplest  InputSameDT=off
  GreaterThan1 : RelationalOperator  Operator=<=  OutDataTypeStr=boolean  RndMeth=Simplest  InputSameDT=off
  Scope : Scope  NumInputPorts=2
      settings: ActiveDisplayYMinimum=-3.73705  ActiveDisplayYMaximum=3.74854  DataLoggingVariableName=ScopeData2
  Sine Wave : Sin  Amplitude=3  Frequency=3  SampleTime=0
  Switch : Switch  Criteria=u2 > Threshold  SaturateOnIntegerOverflow=off  InputSameDT=off
  Switch2 : Switch  Criteria=u2 > Threshold  SaturateOnIntegerOverflow=off  InputSameDT=off
  Unit Delay : UnitDelay  SampleTime=-1  HasFrameUpgradeWarning=on
  wires:
  Unit Delay/1 -> Switch2/3
  Constant3/1 -> Switch2/1
  Switch/1 -> Unit Delay/1, Scope/2
  Switch2/1 -> Switch/3
  Constant2/1 -> Switch/1
  Constant1/1 -> GreaterThan1/2
  Sine Wave/1 -> Scope/1, GreaterThan/1, GreaterThan1/1
  Constant/1 -> GreaterThan/2
  GreaterThan/1 -> Switch/2
  GreaterThan1/1 -> Switch2/2

== system BASIC_PRACTICES/PRACTICES/Simulink/timer/ON_OFF_DELAY_ONE_STEP/OFF_DELAY ==
  Constant1 : Constant
  GreaterThan : RelationalOperator  Operator=<  OutDataTypeStr=boolean  RndMeth=Simplest  InputSameDT=off
  Pulse Generator : DiscretePulseGenerator  PulseType=Time based  PulseWidth=50  PhaseDelay=1
  Scope : Scope  NumInputPorts=2
      settings: ActiveDisplayYMinimum=-0.125  ActiveDisplayYMaximum=1.125
  Switch : Switch  Criteria=u2 > Threshold  SaturateOnIntegerOverflow=off  InputSameDT=off
  Unit Delay1 : UnitDelay  SampleTime=-1  HasFrameUpgradeWarning=on
  wires:
  Constant1/1 -> GreaterThan/2
  Switch/1 -> Scope/2
  GreaterThan/1 -> Switch/2
  Pulse Generator/1 -> Scope/1, Unit Delay1/1, Switch/3, GreaterThan/1
  Unit Delay1/1 -> Switch/1

== system BASIC_PRACTICES/PRACTICES/Simulink/timer/ON_OFF_DELAY_ONE_STEP/ON_DELAY ==
  Constant1 : Constant
  GreaterThan : RelationalOperator  Operator=<  OutDataTypeStr=boolean  RndMeth=Simplest  InputSameDT=off
  Pulse Generator : DiscretePulseGenerator  PulseType=Time based  PulseWidth=50  PhaseDelay=1
  Scope : Scope  NumInputPorts=2
      settings: ActiveDisplayYMinimum=-0.125  ActiveDisplayYMaximum=1.125  DataLoggingVariableName=ScopeData5
  Switch : Switch  Criteria=u2 > Threshold  SaturateOnIntegerOverflow=off  InputSameDT=off
  Unit Delay : UnitDelay  SampleTime=-1  HasFrameUpgradeWarning=on
  wires:
  Pulse Generator/1 -> Scope/1, Switch/1, Unit Delay/1, GreaterThan/1
  Constant1/1 -> GreaterThan/2
  Unit Delay/1 -> Switch/3
  GreaterThan/1 -> Switch/2
  Switch/1 -> Scope/2

== stateflow chart BASIC_PRACTICES/PRACTICES/Stateflow/For_loop/Chart1 ==
  (default) -> (junction 3) : {i=1;
      | out=0;}
  (junction 3) -> (junction 4) [order 1] : [i<=10]
  (junction 4) -> (junction 6) : {out=out+i;}
  (junction 6) -> (junction 3) : {i=i+1;}
  (junction 3) -> (junction 5) [order 2]
  data: out output =0; i local

== stateflow chart BASIC_PRACTICES/TO_STUDY/Chart ==
  state ?
  state ?
  state ggh
    en:bnb
    (history)
    state ?
    state ?
    (default) -> ggh.?
    ggh.? -> ggh.?
    ggh.? -> ggh.?
  state bnb [function]
    (default) -> (junction 12)
  state ?
  state ? [function]
  state ?
  ? -> ?
  (default) -> ggh
  ggh -> ? [order 2]
  ? -> ggh [order 2]
  ggh -> ? [order 3]
  ? -> ? [order 1]
  (junction 3) -> ggh
  ggh -> (junction 3) [order 1]
  data: sf_internal_action_state_placeholder_data local double size=1 =0; sf_internal_action_state_placeholder_data local double size=1 =0
  function ?:
    | function
  function ?:
    | function ?

== matlab function BASIC_PRACTICES/PRACTICES/Subsystem/BY_MATLAB_function/MATLAB Function ==
  data: n input; y output
function y = factorial(n)
y = 1;
for i = 1:n
    y = y * i;
end
end

== stateflow chart BASIC_PRACTICES/PRACTICES/Stateflow/counter/Chart ==
  state stateA
    entry:
    during:
    z=z+1
  state stateB
    entry:
    during:
    z=z-1
  (default) -> stateA
  stateA -> stateB : [z==5]
  stateB -> stateA : [z==0]
  data: z output =0

== matlab function BASIC_PRACTICES/PRACTICES/Simulink/Matlab_function_block/MATLAB Function ==
  data: u input; y output
function y = sum(u)
if (u>2.5)
    y=1;
elseif (u>=0 && u<=2.5)
    y=0;
else
    y= -1;
end

== stateflow chart BASIC_PRACTICES/PRACTICES/Stateflow/if_else/Chart ==
  (default) -> (junction 7) : % h
  (junction 7) -> (junction 8) [order 1] : [h>0]
  (junction 7) -> (junction 9) [order 2] : {y=h-2;}
  (junction 8) -> (junction 10) : {y=h+2;}
  (junction 10) -> (junction 9)
  (junction 9) -> (junction 11)
  data: h input; y output

== stateflow chart BASIC_PRACTICES/PRACTICES/Stateflow/delay_wo_delay_block/Chart ==
  (default) -> (junction 5)
  (junction 5) -> (junction 1)
  (junction 1) -> (junction 2) [order 1] : [t==0]
  (junction 1) -> (junction 3) [order 2] : {out=oldIn;
      | oldValue=in;}
  (junction 2) -> (junction 4) : {out= inVal;
      | oldValue=in;
      | out=oldIn;}
  (junction 4) -> (junction 3)
  data: inVal input uint16; out output uint16; oldIn input uint16; t input uint16; in input uint16; oldValue output uint16

== stateflow chart BASIC_PRACTICES/PRACTICES/Stateflow/For_loop/Chart ==
  (default) -> (junction 3) : {i=1;
      | out=0;}
  (junction 7) -> (junction 4) [order 1] : [i<=10]
  (junction 4) -> (junction 6) : {out=out+i;}
  (junction 3) -> (junction 7) [order 1] : [en==1]
  (junction 6) -> (junction 7) : {i=i+1;}
  (junction 3) -> (junction 5) [order 2]
  (junction 7) -> (junction 14) [order 2]
  (junction 14) -> (junction 5)
  data: out output; i local; en input
